simulink model "ThdRwRtStBkReclnCtrl"  (R2024b)
settings: Solver=FixedStepDiscrete  StartTime=0.0  StopTime=10.0  FixedStep=0.01  RelTol=1e-3
undefined symbols (not defined in the file or in its folder): KeSMSuMdMotFinshdTm_Val, KeSMSuMdRetryTm1_Val, KeSMSuModeReqDurgTm_Val
libraries: StCtrlLib x1
settings Model: Creator=sn2xws  LastModifiedBy=sn55gm
settings SolverCC: AlgebraicLoopSolver=TrustRegion
settings DataIOCC: SaveFormat=StructureWithTime  ReturnWorkspaceOutputs=off
settings OptimizationCC: DefaultParameterBehavior=Inlined  EnhancedBackFolding=on  PassReuseOutputArgsAs=Individual arguments  ZeroExternalMemoryAtStartup=off  ZeroInternalMemoryAtStartup=off  OptimizeBlockOrder=speed  DifferentSizesBufferReuse=on  OptimizationCustomize=off  EfficientTunableParamExpr=on
settings DebuggingCC: ParameterTunabilityLossMsg=error  UnconnectedInputMsg=warning  UnconnectedOutputMsg=warning  UnconnectedLineMsg=warning  ArithmeticOperatorsInVariantConditions=warning
settings ModelReferenceCC: EnableRefExpFcnMdlSchedulingChecks=on  ModelReferenceNumInstancesAllowed=Single
settings SFSimCC: MATLABDynamicMemAlloc=off  CustomCodeUndefinedFunction=UseInterfaceOnly
settings RTWCC: Description=AUTOSAR  SystemTargetFile=autosar.tlc  GenCodeOnly=on  TemplateMakefile=ert_default_tmf  GenerateReport=on  IncludeHyperlinkInReport=on  LaunchReport=on  DataTypeReplacement=CDataTypesFixedWidth  GenerateTraceInfo=on  GenerateTraceReport=on  GenerateTraceReportSl=on  GenerateTraceReportSf=on  GenerateTraceReportEml=on  GPUComputeCapability=3.5
settings CodeAppCC: ForceParamTrailComments=on  IgnoreCustomStorageClasses=off  OperatorAnnotations=on  SimulinkDataObjDesc=on  SFDataObjDesc=on  InsertBlockDesc=on
settings STFCustomTargetCC: TargetLangStandard=C99 (ISO)  MultiwordLength=256  ParMdlRefBuildCompliant=on  CompOptLevelCompliant=on  IncludeMdlTerminateFcn=off  CombineOutputUpdateFcns=on  SuppressErrorStatus=on  ERTCustomFileBanners=on  SupportNonFinite=off  SupportComplex=off  SupportContinuousTime=off  SupportNonInlinedSFcns=off  RemoveResetFunc=on  MATLABClassNameForMDSCustomization=Simulink.SoftwareTarget.ERTCustomization  AutosarCompliant=on  UseToolchainInfoCompliant=on  LookupTableObjectStructAxisOrder=2,1,3,4,...  LUTObjectStructOrderEvenSpacing=Size,Table,Breakpoints  SystemTargetFile=autosar.tlc
settings ERTTargetCC: TargetLangStandard=C99 (ISO)  ConcurrentExecutionCompliant=off  IncludeMdlTerminateFcn=off  SuppressErrorStatus=on  SupportNonFinite=off  SupportComplex=off  ModelStepFunctionPrototypeControlCompliant=off  CPPClassGenCompliant=off  AutosarCompliant=on  LookupTableObjectStructAxisOrder=2,1,3,4,...  LUTObjectStructOrderEvenSpacing=Size,Table,Breakpoints  ERTCustomFileTemplate=example_file_process.tlc  ERTFilePackagingFormat=Compact  BooleanTrueId=TRUE  BooleanFalseId=FALSE  DynamicArrayContainerType=coder::array

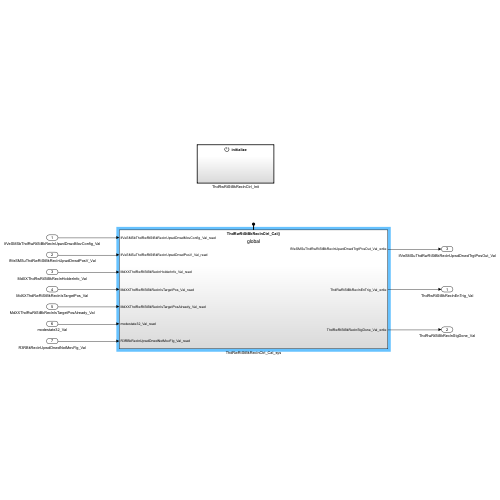
[thumbnail: Simulink's stored preview of the top-level diagram]
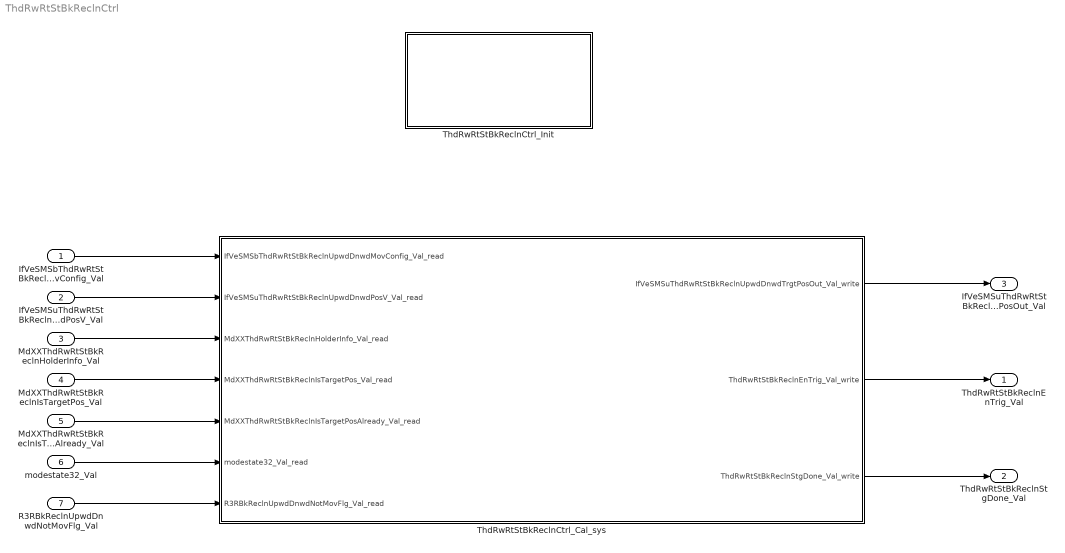
== system ThdRwRtStBkReclnCtrl ==
  IfVeSMSbThdRwRtStBkReclnUpwdDnwdMovConfig_Val : Inport  OutDataTypeStr=boolean  PortDimensions=1
  IfVeSMSuThdRwRtStBkReclnUpwdDnwdPosV_Val : Inport  Port=2  OutDataTypeStr=boolean  PortDimensions=1
  MdXXThdRwRtStBkReclnHolderInfo_Val : Inport  Port=3  OutDataTypeStr=uint32  PortDimensions=1
  MdXXThdRwRtStBkReclnIsTargetPos_Val : Inport  Port=4  OutDataTypeStr=uint32  PortDimensions=1
  MdXXThdRwRtStBkReclnIsTargetPosAlready_Val : Inport  Port=5  OutDataTypeStr=uint32  PortDimensions=1
  modestate32_Val : Inport  Port=6  OutDataTypeStr=uint32  PortDimensions=1
  R3RBkReclnUpwdDnwdNotMovFlg_Val : Inport  Port=7  OutDataTypeStr=boolean  PortDimensions=1
  ThdRwRtStBkReclnCtrl_Cal_sys : Subsystem
  ThdRwRtStBkReclnCtrl_Init : Subsystem
  ThdRwRtStBkReclnEnTrig_Val : Outport  OutDataTypeStr=boolean  PortDimensions=1  VectorParamsAs1DForOutWhenUnconnected=off
  ThdRwRtStBkReclnStgDone_Val : Outport  Port=2  OutDataTypeStr=boolean  PortDimensions=1  VectorParamsAs1DForOutWhenUnconnected=off
  IfVeSMSuThdRwRtStBkReclnUpwdDnwdTrgtPosOut_Val : Outport  Port=3  OutDataTypeStr=boolean  PortDimensions=1  VectorParamsAs1DForOutWhenUnconnected=off
  wires:
  IfVeSMSbThdRwRtStBkReclnUpwdDnwdMovConfig_Val/1 -> ThdRwRtStBkReclnCtrl_Cal_sys/1(IfVeSMSbThdRwRtStBkReclnUpwdDnwdMovConfig_Val_read)
  IfVeSMSuThdRwRtStBkReclnUpwdDnwdPosV_Val/1 -> ThdRwRtStBkReclnCtrl_Cal_sys/2(IfVeSMSuThdRwRtStBkReclnUpwdDnwdPosV_Val_read)
  MdXXThdRwRtStBkReclnHolderInfo_Val/1 -> ThdRwRtStBkReclnCtrl_Cal_sys/3(MdXXThdRwRtStBkReclnHolderInfo_Val_read)
  MdXXThdRwRtStBkReclnIsTargetPos_Val/1 -> ThdRwRtStBkReclnCtrl_Cal_sys/4(MdXXThdRwRtStBkReclnIsTargetPos_Val_read)
  MdXXThdRwRtStBkReclnIsTargetPosAlready_Val/1 -> ThdRwRtStBkReclnCtrl_Cal_sys/5(MdXXThdRwRtStBkReclnIsTargetPosAlready_Val_read)
  modestate32_Val/1 -> ThdRwRtStBkReclnCtrl_Cal_sys/6(modestate32_Val_read)
  R3RBkReclnUpwdDnwdNotMovFlg_Val/1 -> ThdRwRtStBkReclnCtrl_Cal_sys/7(R3RBkReclnUpwdDnwdNotMovFlg_Val_read)
  ThdRwRtStBkReclnCtrl_Cal_sys/1(IfVeSMSuThdRwRtStBkReclnUpwdDnwdTrgtPosOut_Val_write) -> IfVeSMSuThdRwRtStBkReclnUpwdDnwdTrgtPosOut_Val/1
  ThdRwRtStBkReclnCtrl_Cal_sys/2(ThdRwRtStBkReclnEnTrig_Val_write) -> ThdRwRtStBkReclnEnTrig_Val/1
  ThdRwRtStBkReclnCtrl_Cal_sys/3(ThdRwRtStBkReclnStgDone_Val_write) -> ThdRwRtStBkReclnStgDone_Val/1

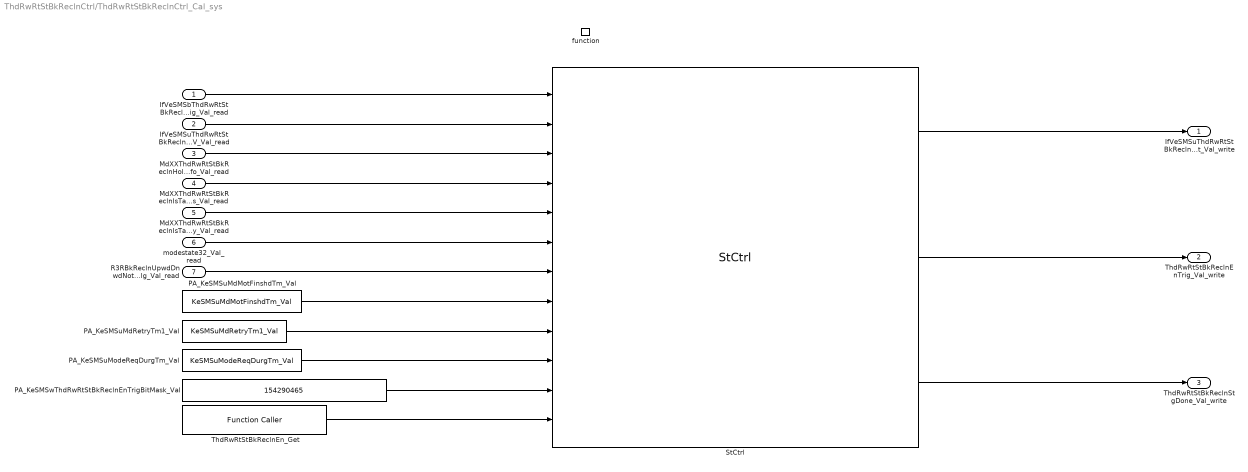
== system ThdRwRtStBkReclnCtrl/ThdRwRtStBkReclnCtrl_Cal_sys ==
  IfVeSMSbThdRwRtStBkReclnUpwdDnwdMovConfig_Val_read : Inport
  IfVeSMSuThdRwRtStBkReclnUpwdDnwdPosV_Val_read : Inport  Port=2
  MdXXThdRwRtStBkReclnHolderInfo_Val_read : Inport  Port=3
  MdXXThdRwRtStBkReclnIsTargetPos_Val_read : Inport  Port=4
  MdXXThdRwRtStBkReclnIsTargetPosAlready_Val_read : Inport  Port=5
  modestate32_Val_read : Inport  Port=6
  R3RBkReclnUpwdDnwdNotMovFlg_Val_read : Inport  Port=7
  function : TriggerPort  TriggerType=function-call  IsSimulinkFunction=on  FunctionName=ThdRwRtStBkReclnCtrl_Cal  VariantControl=(inherit)
  PA_KeSMSuMdMotFinshdTm_Val : Constant  Value=KeSMSuMdMotFinshdTm_Val
  PA_KeSMSuMdRetryTm1_Val : Constant  Value=KeSMSuMdRetryTm1_Val
  PA_KeSMSuModeReqDurgTm_Val : Constant  Value=KeSMSuModeReqDurgTm_Val
  PA_KeSMSwThdRwRtStBkReclnEnTrigBitMask_Val : Constant  Value=154290465  OutDataTypeStr=uint32
  StCtrl : StCtrlLib/StCtrl  SystemSampleTime=-1  VariantActivationTime=update diagram  AllowFlexibleInterface=on  Latency=0  AutoFrameSizeCalculation=off
  ThdRwRtStBkReclnEn_Get : FunctionCaller  FunctionPrototype=data = ThdRwRtStBkReclnEn_Get()  InputArgumentSpecifications=<Enter example>  OutputArgumentSpecifications=uint32(1)
  IfVeSMSuThdRwRtStBkReclnUpwdDnwdTrgtPosOut_Val_write : Outport  VectorParamsAs1DForOutWhenUnconnected=off
      settings: EnsureOutportIsVirtual=on
  ThdRwRtStBkReclnEnTrig_Val_write : Outport  Port=2  VectorParamsAs1DForOutWhenUnconnected=off
      settings: EnsureOutportIsVirtual=on
  ThdRwRtStBkReclnStgDone_Val_write : Outport  Port=3  VectorParamsAs1DForOutWhenUnconnected=off
      settings: EnsureOutportIsVirtual=on
  wires:
  StCtrl/1 -> IfVeSMSuThdRwRtStBkReclnUpwdDnwdTrgtPosOut_Val_write/1
  StCtrl/2 -> ThdRwRtStBkReclnEnTrig_Val_write/1
  StCtrl/3 -> ThdRwRtStBkReclnStgDone_Val_write/1
  PA_KeSMSwThdRwRtStBkReclnEnTrigBitMask_Val/1 -> StCtrl/11
  ThdRwRtStBkReclnEn_Get/1 -> StCtrl/12
  PA_KeSMSuMdMotFinshdTm_Val/1 -> StCtrl/8
  PA_KeSMSuModeReqDurgTm_Val/1 -> StCtrl/10
  PA_KeSMSuMdRetryTm1_Val/1 -> StCtrl/9
  IfVeSMSbThdRwRtStBkReclnUpwdDnwdMovConfig_Val_read/1 -> StCtrl/1
  IfVeSMSuThdRwRtStBkReclnUpwdDnwdPosV_Val_read/1 -> StCtrl/2
  MdXXThdRwRtStBkReclnHolderInfo_Val_read/1 -> StCtrl/3
  MdXXThdRwRtStBkReclnIsTargetPos_Val_read/1 -> StCtrl/4
  MdXXThdRwRtStBkReclnIsTargetPosAlready_Val_read/1 -> StCtrl/5
  modestate32_Val_read/1 -> StCtrl/6
  R3RBkReclnUpwdDnwdNotMovFlg_Val_read/1 -> StCtrl/7

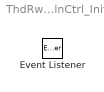
== system ThdRwRtStBkReclnCtrl/ThdRwRtStBkReclnCtrl_Init ==
  Event Listener : EventListener  EventName=reset
